simulink model "possible_sketch"  (R2020a)
settings: Solver=FixedStepAuto  StartTime=0.0  StopTime=2000.0  RelTol=1e-3  EnableMultiTasking=on
libraries: simulink x2
settings Model: SimulationMode=external  ExtModeTrigDuration=2  Creator=bengt  LastModifiedBy=bengt
settings DataIOCC: DSMLogging=off  ReturnWorkspaceOutputs=off
settings OptimizationCC: DefaultParameterBehavior=Inlined  DefaultUnderspecifiedDataType=single  LifeSpan=1  MaxStackSize=64  EfficientTunableParamExpr=on
settings DebuggingCC: PregeneratedLibrarySubsystemCodeDiagnostic=none  SFUnexpectedBacktrackingDiag=warning  SFNoUnconditionalDefaultTransitionDiag=warning  SFExecutionAtInitializationDiag=none  ArithmeticOperatorsInVariantConditions=warning
settings HardwareCC: ProdBitPerInt=16  ProdBitPerPointer=16  ProdBitPerSizeT=16  ProdBitPerPtrDiffT=16  ProdLargestAtomicFloat=None  ProdWordSize=16  ProdHWDeviceType=STMicroelectronics->ST10/Super10
settings ModelReferenceCC: UpdateModelReferenceTargets=Force  PropagateSignalLabelsOutOfModel=off
settings SFSimCC: SimUseLocalCustomCode=off  MATLABDynamicMemAlloc=off  CustomCodeUndefinedFunction=UseInterfaceOnly
settings RTWCC: SystemTargetFile=ert.tlc  TemplateMakefile=ert_default_tmf  GenerateReport=on  RTWUseLocalCustomCode=off  Toolchain=Arduino AVR v1.6.1  BuildConfiguration=Faster Runs  IncludeHyperlinkInReport=on  LaunchReport=on  PortableWordSizes=on  GenerateTraceInfo=on  GenerateTraceReport=on  GenerateTraceReportSl=on  GenerateTraceReportSf=on  GenerateTraceReportEml=on  GenerateCodeMetricsReport=on
settings CodeAppCC: ForceParamTrailComments=on  IgnoreCustomStorageClasses=off  OperatorAnnotations=on  SimulinkDataObjDesc=on  SFDataObjDesc=on  MATLABFcnDesc=on  InsertBlockDesc=on  StateflowObjectComments=on  MATLABSourceComments=on
settings ERTTargetCC: MultiwordLength=2048  SupportContinuousTime=on  SupportVariableSizeSignals=on  ERTCustomFileTemplate=example_file_process.tlc  IndentStyle=Allman  IndentSize=4
settings ConfigComp: CovMetricSettings=dw  CovHtmlReporting=on  CovSaveCumulativeToWorkspaceVar=on  CovSaveSingleToWorkspaceVar=on  CovExternalEMLEnable=off

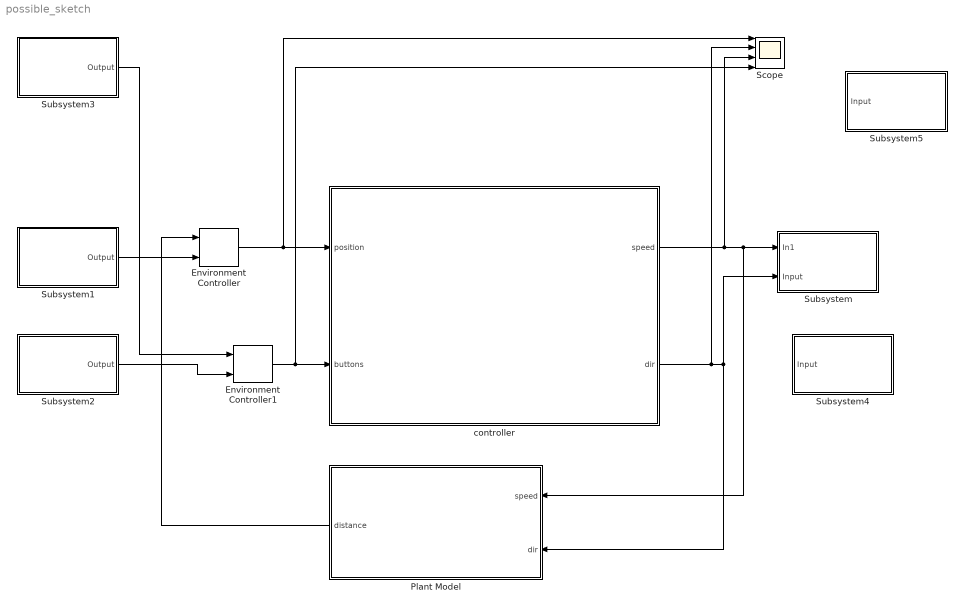
== system possible_sketch ==
  Environment Controller : simulink/Signal Routing/Environment Controller
      settings: SourceProductBaseCode=SL
  Environment Controller1 : simulink/Signal Routing/Environment Controller
      settings: SourceProductBaseCode=SL
  Plant Model : Subsystem
      mask Display: disp('Simulink Model of Elevator Dynamics')
  Scope : Scope  NumInputPorts=4
  Subsystem : Subsystem
      mask Display: disp('Driver Block for Motor')
  Subsystem1 : Subsystem
      mask Display: disp('Driver Block for Sensor')
  Subsystem2 : Subsystem
      mask Display: disp('Button Driver Block(s)')
  Subsystem3 : Subsystem
      mask Display: disp('Simulink Buttons')
  Subsystem4 : Subsystem
      mask Display: disp('Lamps Driver Block(s)')
  Subsystem5 : Subsystem
      mask Display: disp('Simulink Lamps')
  controller : Stateflow chart  TreatAsAtomicUnit=on  mask{GroundHeight=100, FloorHeight=180, FloorTolerance=5, AscendingRate=255.000, DescendingRate=200, FloorDelay=2000}
      mask prompts: GroundHeight "Ground Height (mm)"; FloorHeight "Floor Height (mm)"; FloorTolerance "Floor Tolerance (mm)"; AscendingRate "Ascending Rate"; DescendingRate "Descending Rate"; FloorDelay "Delay on the floors (msec)"
  wires:
  Subsystem1/1(Output) -> Environment Controller/2
  Plant Model/1(distance) -> Environment Controller/1
  Environment Controller/1 -> controller/1(position), Scope/1
  controller/1(speed) -> Scope/3, Subsystem/1(In1), Plant Model/1(speed)
  controller/2(dir) -> Scope/2, Subsystem/2(Input), Plant Model/2(dir)
  Environment Controller1/1 -> Scope/4, controller/2(buttons)
  Subsystem2/1(Output) -> Environment Controller1/2
  Subsystem3/1(Output) -> Environment Controller1/1

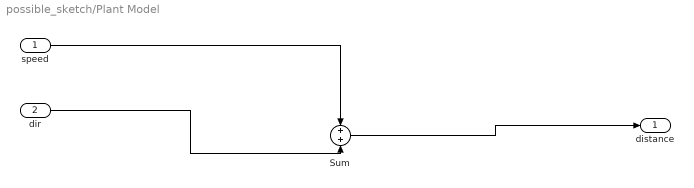
== system possible_sketch/Plant Model ==
  speed : Inport
  dir : Inport  Port=2
  Sum : Sum
  distance : Outport  VectorParamsAs1DForOutWhenUnconnected=off
  wires:
  speed/1 -> Sum/1
  dir/1 -> Sum/2
  Sum/1 -> distance/1

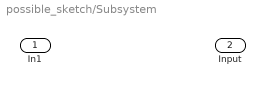
== system possible_sketch/Subsystem ==
  In1 : Inport
  Input : Inport  Port=2

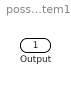
== system possible_sketch/Subsystem1 ==
  Output : Outport  VectorParamsAs1DForOutWhenUnconnected=off

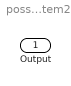
== system possible_sketch/Subsystem2 ==
  Output : Outport  VectorParamsAs1DForOutWhenUnconnected=off

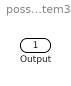
== system possible_sketch/Subsystem3 ==
  Output : Outport  VectorParamsAs1DForOutWhenUnconnected=off

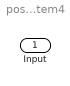
== system possible_sketch/Subsystem4 ==
  Input : Inport

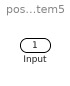
== system possible_sketch/Subsystem5 ==
  Input : Inport

== stateflow chart possible_sketch/controller ==
  settings: sampleTime=0.1
  state S1
  state S2
  (default) -> S1
  S1 -> S2 : [0]
  S2 -> S1 : [0]
  data: goto local boolean size=4 =[1 0 0 0]; position input uint16 size=1; speed output uint8 size=1; TargetsLower constant double size=4 =([0:3] .* FloorHeight) + GroundHeight - FloorTolerance; TargetsUpper constant double size=4 =([0:3] .* FloorHeight) + GroundHeight + FloorTolerance; SpeedUp constant double size=1 =AscendingRate; SpeedDown constant double size=1 =DescendingRate; dir output boolean; Targets constant double size=4 =([0:3] .* FloorHeight) + GroundHeight; dirPrev local boolean; floor local double; buttons input boolean size=4; Delay constant double =FloorDelay
